simulink model "Temporal7_2018a"  (R2018a)
settings: Solver=VariableStepAuto  StartTime=0.0  StopTime=0.5  RelTol=1e-3
settings Model: Creator=86188  LastModifiedBy=bzhan

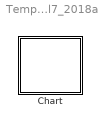
== system Temporal7_2018a ==
  Chart : Stateflow chart  TreatAsAtomicUnit=on

== stateflow chart Temporal7_2018a/Chart ==
  settings: updateMethod=DISCRETE  sampleTime=0.1
  state A
    en:f("en_A");
  state B
    en:f("en_B");
  (default) -> A
  A -> B [order 1] : after(1,tick)
  A -> A [order 2]
  B -> A
  data: s function_input; x local
  function f(s):
    | function f(s)
    |   fprintf(s+"\n");
